simulink model "w3_warplab_buffers"  (Simulink 7.7)
settings: Solver=VariableStepDiscrete  SolverMode=SingleTasking  StartTime=0.0  StopTime=200000  RelTol=1e-3
InitFcn:
  | w3_warplab_buffers_init
StartFcn:
  | w3_warplab_buffers_init
values from neighbouring files (symbols this model uses):
  NumSamps_Rx_IQ = 2^15    (= 32768)    [w3_warplab_buffers_init.m]
  NumSamps_Rx_RSSI = 2^13    (= 8192)    [w3_warplab_buffers_init.m]
  NumSamps_Tx_IQ = 2^15    (= 32768)    [w3_warplab_buffers_init.m]
undefined symbols (not defined in the file or in its folder): gcbh, xlBlockLoadCallback, xlGetNormalizedPeriod
libraries: xbsIndex_r4 x1266, xbsEDKLib_r4 x1
(part 7 of 9)

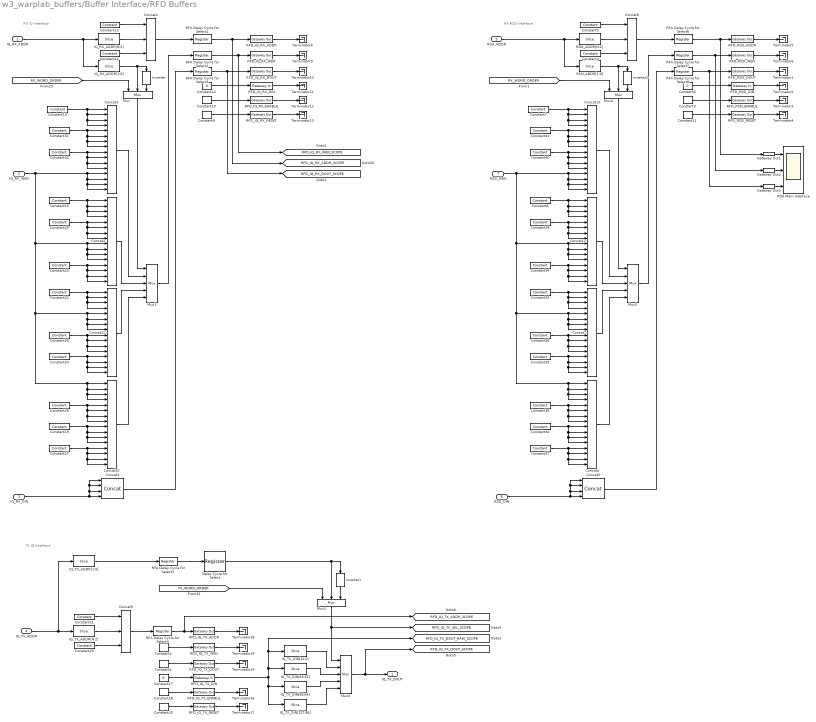
== system w3_warplab_buffers/Buffer Interface/RFD Buffers ==
  note: RX IQ Interface
  note: TX IQ Interface
  note: RX RSSI Interface
  IQ_RX_ADDR : Inport
  IQ_RX_WEN : Inport  Port=2
  IQ_RX_DIN : Inport  Port=3
  IQ_TX_ADDR : Inport  Port=4
  RSSI_ADDR : Inport  Port=5
  RSSI_DIN : Inport  Port=6
  RSSI_WEN : Inport  Port=7
  Concat1 : xbsIndex_r4/Concat  num_inputs=4  dbl_ovrd=off  block_type=concat
  Concat{2..3,6..7,10..13} (8 alike) : xbsIndex_r4/Concat  num_inputs=16  dbl_ovrd=off  block_type=concat
  Concat4 : xbsIndex_r4/Concat  num_inputs=3  dbl_ovrd=off  block_type=concat
  Concat5 : xbsIndex_r4/Concat  num_inputs=4  dbl_ovrd=off  block_type=concat
  Concat8 : xbsIndex_r4/Concat  num_inputs=3  dbl_ovrd=off  block_type=concat
  Concat9 : xbsIndex_r4/Concat  num_inputs=3  dbl_ovrd=off  block_type=concat
  Constant1 : xbsIndex_r4/Constant  const=0  gui_display_data_type=Fixed-point  arith_type=Unsigned  n_bits=128  bin_pt=0  preci_type=Single  exp_width=8  frac_width=24  explicit_period=off  period=1  equ=P=C  opselect=C  inp2=PCIN>>17  opr=+  inp1=P  carry=CIN  dbl_ovrd=off  block_type=constant
      settings: block_version=10.1.2
  Constant10 : xbsIndex_r4/Constant  const=1  gui_display_data_type=Boolean  arith_type=Boolean  n_bits=32  bin_pt=0  preci_type=Single  exp_width=8  frac_width=24  explicit_period=off  period=1  equ=P=C  opselect=C  inp2=PCIN>>17  opr=+  inp1=P  carry=CIN  dbl_ovrd=off  block_type=constant
      settings: block_version=10.1.2
  Constant11 : xbsIndex_r4/Constant  const=0  gui_display_data_type=Boolean  arith_type=Boolean  n_bits=32  bin_pt=0  preci_type=Single  exp_width=8  frac_width=24  explicit_period=off  period=1  equ=P=C  opselect=C  inp2=PCIN>>17  opr=+  inp1=P  carry=CIN  dbl_ovrd=off  block_type=constant
      settings: block_version=10.1.2
  Constant12 : xbsIndex_r4/Constant  const=0  gui_display_data_type=Fixed-point  arith_type=Unsigned  n_bits=4  bin_pt=0  preci_type=Single  exp_width=8  frac_width=24  explicit_period=off  period=1  equ=P=C  opselect=C  inp2=PCIN>>17  opr=+  inp1=P  carry=CIN  dbl_ovrd=off  block_type=constant
  Constant13 : xbsIndex_r4/Constant  const=0  gui_display_data_type=Fixed-point  arith_type=Unsigned  n_bits=30 - ceil(log2(NumSamps_Rx_IQ))  bin_pt=0  preci_type=Single  exp_width=8  frac_width=24  explicit_period=off  period=1  equ=P=C  opselect=C  inp2=PCIN>>17  opr=+  inp1=P  carry=CIN  dbl_ovrd=off  block_type=constant
  Constant14 : Constant  Value=0
  Constant{7..8,15..16,19,22..24,26..41} (24 alike) : xbsIndex_r4/Constant  const=0  gui_display_data_type=Boolean  arith_type=Boolean  n_bits=1  bin_pt=0  preci_type=Single  exp_width=8  frac_width=24  explicit_period=off  period=1  equ=P=C  opselect=C  inp2=PCIN>>17  opr=+  inp1=P  carry=CIN  dbl_ovrd=off  block_type=constant
  Constant17 : Constant  Value=0
  Constant18 : xbsIndex_r4/Constant  const=1  gui_display_data_type=Boolean  arith_type=Boolean  n_bits=32  bin_pt=0  preci_type=Single  exp_width=8  frac_width=24  explicit_period=off  period=1  equ=P=C  opselect=C  inp2=PCIN>>17  opr=+  inp1=P  carry=CIN  dbl_ovrd=off  block_type=constant
      settings: block_version=10.1.2
  Constant2 : xbsIndex_r4/Constant  const=0  gui_display_data_type=Fixed-point  arith_type=Unsigned  n_bits=16  bin_pt=0  preci_type=Single  exp_width=8  frac_width=24  explicit_period=off  period=1  equ=P=C  opselect=C  inp2=PCIN>>17  opr=+  inp1=P  carry=CIN  dbl_ovrd=off  block_type=constant
      settings: block_version=10.1.2
  Constant20 : xbsIndex_r4/Constant  const=0  gui_display_data_type=Fixed-point  arith_type=Unsigned  n_bits=4  bin_pt=0  preci_type=Single  exp_width=8  frac_width=24  explicit_period=off  period=1  equ=P=C  opselect=C  inp2=PCIN>>17  opr=+  inp1=P  carry=CIN  dbl_ovrd=off  block_type=constant
  Constant21 : xbsIndex_r4/Constant  const=0  gui_display_data_type=Fixed-point  arith_type=Unsigned  n_bits=30 - ceil(log2(NumSamps_Tx_IQ))  bin_pt=0  preci_type=Single  exp_width=8  frac_width=24  explicit_period=off  period=1  equ=P=C  opselect=C  inp2=PCIN>>17  opr=+  inp1=P  carry=CIN  dbl_ovrd=off  block_type=constant
  Constant25 : xbsIndex_r4/Constant  const=0  gui_display_data_type=Boolean  arith_type=Boolean  n_bits=32  bin_pt=0  preci_type=Single  exp_width=8  frac_width=24  explicit_period=off  period=1  equ=P=C  opselect=C  inp2=PCIN>>17  opr=+  inp1=P  carry=CIN  dbl_ovrd=off  block_type=constant
      settings: block_version=10.1.2
  Constant3 : xbsIndex_r4/Constant  const=1  gui_display_data_type=Boolean  arith_type=Boolean  n_bits=32  bin_pt=0  preci_type=Single  exp_width=8  frac_width=24  explicit_period=off  period=1  equ=P=C  opselect=C  inp2=PCIN>>17  opr=+  inp1=P  carry=CIN  dbl_ovrd=off  block_type=constant
      settings: block_version=10.1.2
  Constant4 : xbsIndex_r4/Constant  const=0  gui_display_data_type=Fixed-point  arith_type=Unsigned  n_bits=4  bin_pt=0  preci_type=Single  exp_width=8  frac_width=24  explicit_period=off  period=1  equ=P=C  opselect=C  inp2=PCIN>>17  opr=+  inp1=P  carry=CIN  dbl_ovrd=off  block_type=constant
  Constant5 : xbsIndex_r4/Constant  const=0  gui_display_data_type=Fixed-point  arith_type=Unsigned  n_bits=31 - ceil(log2(NumSamps_Rx_RSSI))  bin_pt=0  preci_type=Single  exp_width=8  frac_width=24  explicit_period=off  period=1  equ=P=C  opselect=C  inp2=PCIN>>17  opr=+  inp1=P  carry=CIN  dbl_ovrd=off  block_type=constant
  Constant6 : Constant  Value=0
  Constant9 : xbsIndex_r4/Constant  const=0  gui_display_data_type=Boolean  arith_type=Boolean  n_bits=32  bin_pt=0  preci_type=Single  exp_width=8  frac_width=24  explicit_period=off  period=1  equ=P=C  opselect=C  inp2=PCIN>>17  opr=+  inp1=P  carry=CIN  dbl_ovrd=off  block_type=constant
      settings: block_version=10.1.2
  Delay Cycle for Select : xbsIndex_r4/Register  init=0  rst=off  en=off  dbl_ovrd=off  block_type=register
  Gateway Out1 : xbsIndex_r4/Gateway Out  inherit_from_input=off  hdl_port=off  timing_constraint=None  locs_specified=off  LOCs={}  UseAsDAC=off  DACChannel='1'  block_type=gatewayout
      settings: infoedit="Gateway out block.  Converts Xilinx fixed point inputs into ouputs of type Simulink integer, double, or fixed point.<P><P>Hardware notes:  In hardware these blocks become top level output ports or are discarded, depending on how they are configured."  block_version=10.1.2
  Gateway Out2 : xbsIndex_r4/Gateway Out  inherit_from_input=off  hdl_port=off  timing_constraint=None  locs_specified=off  LOCs={}  UseAsDAC=off  DACChannel='1'  block_type=gatewayout
      settings: infoedit="Gateway out block.  Converts Xilinx fixed point inputs into ouputs of type Simulink integer, double, or fixed point.<P><P>Hardware notes:  In hardware these blocks become top level output ports or are discarded, depending on how they are configured."  block_version=10.1.2
  Gateway Out3 : xbsIndex_r4/Gateway Out  inherit_from_input=off  hdl_port=off  timing_constraint=None  locs_specified=off  LOCs={}  UseAsDAC=off  DACChannel='1'  block_type=gatewayout
      settings: infoedit="Gateway out block.  Converts Xilinx fixed point inputs into ouputs of type Simulink integer, double, or fixed point.<P><P>Hardware notes:  In hardware these blocks become top level output ports or are discarded, depending on how they are configured."  block_version=10.1.2
  IQ_RX_ADDR[1:0] : xbsIndex_r4/Slice  nbits=2  boolean_output=off  mode=Lower Bit Location + Width  bit1=0  base1=MSB of Input  bit0=0  base0=LSB of Input  dbl_ovrd=off  block_type=slice
  IQ_RX_ADDR[N:2] : xbsIndex_r4/Slice  nbits=ceil(log2(NumSamps_Rx_IQ)) - 2  boolean_output=off  mode=Lower Bit Location + Width  bit1=0  base1=MSB of Input  bit0=2  base0=LSB of Input  dbl_ovrd=off  block_type=slice
  IQ_TX_ADDR[1:0] : xbsIndex_r4/Slice  nbits=2  boolean_output=off  mode=Lower Bit Location + Width  bit1=0  base1=MSB of Input  bit0=0  base0=LSB of Input  dbl_ovrd=off  block_type=slice
  IQ_TX_ADDR[N:2] : xbsIndex_r4/Slice  nbits=ceil(log2(NumSamps_Tx_IQ)) - 2  boolean_output=off  mode=Lower Bit Location + Width  bit1=0  base1=MSB of Input  bit0=2  base0=LSB of Input  dbl_ovrd=off  block_type=slice
  IQ_TX_DIN[127:96] : xbsIndex_r4/Slice  nbits=32  boolean_output=off  mode=Lower Bit Location + Width  bit1=0  base1=MSB of Input  bit0=96  base0=LSB of Input  dbl_ovrd=off  block_type=slice
  IQ_TX_DIN[31:0] : xbsIndex_r4/Slice  nbits=32  boolean_output=off  mode=Lower Bit Location + Width  bit1=0  base1=MSB of Input  bit0=0  base0=LSB of Input  dbl_ovrd=off  block_type=slice
  IQ_TX_DIN[63:32] : xbsIndex_r4/Slice  nbits=32  boolean_output=off  mode=Lower Bit Location + Width  bit1=0  base1=MSB of Input  bit0=32  base0=LSB of Input  dbl_ovrd=off  block_type=slice
  IQ_TX_DIN[95:64] : xbsIndex_r4/Slice  nbits=32  boolean_output=off  mode=Lower Bit Location + Width  bit1=0  base1=MSB of Input  bit0=64  base0=LSB of Input  dbl_ovrd=off  block_type=slice
  Inverter : xbsIndex_r4/Inverter  en=off  latency=0  dbl_ovrd=off  block_type=inv
  Inverter1 : xbsIndex_r4/Inverter  en=off  latency=0  dbl_ovrd=off  block_type=inv
  Inverter2 : xbsIndex_r4/Inverter  en=off  latency=0  dbl_ovrd=off  block_type=inv
  Mux : xbsIndex_r4/Mux  inputs=2  en=off  latency=0  precision=Full  arith_type=Unsigned  n_bits=16  bin_pt=14  quantization=Truncate  overflow=Wrap  dbl_ovrd=off  block_type=mux
  Mux1 : xbsIndex_r4/Mux  inputs=4  en=off  latency=0  precision=Full  arith_type=Unsigned  n_bits=16  bin_pt=14  quantization=Truncate  overflow=Wrap  dbl_ovrd=off  block_type=mux
  Mux2 : xbsIndex_r4/Mux  inputs=2  en=off  latency=0  precision=Full  arith_type=Unsigned  n_bits=16  bin_pt=14  quantization=Truncate  overflow=Wrap  dbl_ovrd=off  block_type=mux
  Mux3 : xbsIndex_r4/Mux  inputs=4  en=off  latency=0  precision=Full  arith_type=Unsigned  n_bits=16  bin_pt=14  quantization=Truncate  overflow=Wrap  dbl_ovrd=off  block_type=mux
  Mux4 : xbsIndex_r4/Mux  inputs=2  en=off  latency=0  precision=Full  arith_type=Unsigned  n_bits=16  bin_pt=14  quantization=Truncate  overflow=Wrap  dbl_ovrd=off  block_type=mux
  Mux5 : xbsIndex_r4/Mux  inputs=4  en=off  latency=0  precision=Full  arith_type=Unsigned  n_bits=16  bin_pt=14  quantization=Truncate  overflow=Wrap  dbl_ovrd=off  block_type=mux
  RFA Delay Cycle for Select{1..8} (8 alike) : xbsIndex_r4/Register  init=0  rst=off  en=off  dbl_ovrd=off  block_type=register
  RFD_IQ_RX_ADDR : xbsIndex_r4/Gateway Out  inherit_from_input=off  hdl_port=on  timing_constraint=None  locs_specified=off  LOCs={}  UseAsDAC=off  DACChannel='1'  block_type=gatewayout
  RFD_IQ_RX_DIN : xbsIndex_r4/Gateway In  gui_display_data_type=Fixed-point  arith_type=Unsigned  n_bits=128  bin_pt=0  preci_type=Single  exp_width=8  frac_width=24  quantization="Round  (unbiased: +/- Inf)"  overflow=Saturate  period=1  dbl_ovrd=off  timing_constraint=None  locs_specified=off  LOCs={}  UseAsADC=off  ADCChannel='1'  inherit_from_input=off  hdl_port=on  block_type=gatewayin
  RFD_IQ_RX_DOUT : xbsIndex_r4/Gateway Out  inherit_from_input=off  hdl_port=on  timing_constraint=None  locs_specified=off  LOCs={}  UseAsDAC=off  DACChannel='1'  block_type=gatewayout
  RFD_IQ_RX_ENABLE : xbsIndex_r4/Gateway Out  inherit_from_input=off  hdl_port=on  timing_constraint=None  locs_specified=off  LOCs={}  UseAsDAC=off  DACChannel='1'  block_type=gatewayout
  RFD_IQ_RX_RESET : xbsIndex_r4/Gateway Out  inherit_from_input=off  hdl_port=on  timing_constraint=None  locs_specified=off  LOCs={}  UseAsDAC=off  DACChannel='1'  block_type=gatewayout
  RFD_IQ_RX_WEN : xbsIndex_r4/Gateway Out  inherit_from_input=off  hdl_port=on  timing_constraint=None  locs_specified=off  LOCs={}  UseAsDAC=off  DACChannel='1'  block_type=gatewayout
  RFD_IQ_TX_ADDR : xbsIndex_r4/Gateway Out  inherit_from_input=off  hdl_port=on  timing_constraint=None  locs_specified=off  LOCs={}  UseAsDAC=off  DACChannel='1'  block_type=gatewayout
  RFD_IQ_TX_DIN : xbsIndex_r4/Gateway In  gui_display_data_type=Fixed-point  arith_type=Unsigned  n_bits=128  bin_pt=0  preci_type=Single  exp_width=8  frac_width=24  quantization="Round  (unbiased: +/- Inf)"  overflow=Saturate  period=1  dbl_ovrd=off  timing_constraint=None  locs_specified=off  LOCs={}  UseAsADC=off  ADCChannel='1'  inherit_from_input=off  hdl_port=on  block_type=gatewayin
  RFD_IQ_TX_DOUT : xbsIndex_r4/Gateway Out  inherit_from_input=off  hdl_port=on  timing_constraint=None  locs_specified=off  LOCs={}  UseAsDAC=off  DACChannel='1'  block_type=gatewayout
  RFD_IQ_TX_ENABLE : xbsIndex_r4/Gateway Out  inherit_from_input=off  hdl_port=on  timing_constraint=None  locs_specified=off  LOCs={}  UseAsDAC=off  DACChannel='1'  block_type=gatewayout
  RFD_IQ_TX_RESET : xbsIndex_r4/Gateway Out  inherit_from_input=off  hdl_port=on  timing_constraint=None  locs_specified=off  LOCs={}  UseAsDAC=off  DACChannel='1'  block_type=gatewayout
  RFD_IQ_TX_WEN : xbsIndex_r4/Gateway Out  inherit_from_input=off  hdl_port=on  timing_constraint=None  locs_specified=off  LOCs={}  UseAsDAC=off  DACChannel='1'  block_type=gatewayout
  RFD_RSSI_ADDR : xbsIndex_r4/Gateway Out  inherit_from_input=off  hdl_port=on  timing_constraint=None  locs_specified=off  LOCs={}  UseAsDAC=off  DACChannel='1'  block_type=gatewayout
  RFD_RSSI_DIN : xbsIndex_r4/Gateway In  gui_display_data_type=Fixed-point  arith_type=Unsigned  n_bits=128  bin_pt=0  preci_type=Single  exp_width=8  frac_width=24  quantization="Round  (unbiased: +/- Inf)"  overflow=Saturate  period=1  dbl_ovrd=off  timing_constraint=None  locs_specified=off  LOCs={}  UseAsADC=off  ADCChannel='1'  inherit_from_input=off  hdl_port=on  block_type=gatewayin
  RFD_RSSI_DOUT : xbsIndex_r4/Gateway Out  inherit_from_input=off  hdl_port=on  timing_constraint=None  locs_specified=off  LOCs={}  UseAsDAC=off  DACChannel='1'  block_type=gatewayout
  RFD_RSSI_ENABLE : xbsIndex_r4/Gateway Out  inherit_from_input=off  hdl_port=on  timing_constraint=None  locs_specified=off  LOCs={}  UseAsDAC=off  DACChannel='1'  block_type=gatewayout
  RFD_RSSI_RESET : xbsIndex_r4/Gateway Out  inherit_from_input=off  hdl_port=on  timing_constraint=None  locs_specified=off  LOCs={}  UseAsDAC=off  DACChannel='1'  block_type=gatewayout
  RFD_RSSI_WEN : xbsIndex_r4/Gateway Out  inherit_from_input=off  hdl_port=on  timing_constraint=None  locs_specified=off  LOCs={}  UseAsDAC=off  DACChannel='1'  block_type=gatewayout
  RSSI Mem Interface : Scope  NumInputPorts=3
      settings: TimeRange=70000  YMin=0~0~0  YMax=1~1~1  SaveName=ScopeData6
  RSSI_ADDR[1:0] : xbsIndex_r4/Slice  nbits=2  boolean_output=off  mode=Lower Bit Location + Width  bit1=0  base1=MSB of Input  bit0=0  base0=LSB of Input  dbl_ovrd=off  block_type=slice
  RSSI_ADDR[N:2] : xbsIndex_r4/Slice  nbits=ceil(log2(NumSamps_Rx_RSSI)) - 3  boolean_output=off  mode=Lower Bit Location + Width  bit1=0  base1=MSB of Input  bit0=2  base0=LSB of Input  dbl_ovrd=off  block_type=slice
  Terminator{1..6,8..14,16..19} (17 alike) : Terminator
  IQ_TX_DOUT : Outport
  tag scope: RFD_IQ_RX_ADDR_SCOPE=global, RFD_IQ_RX_DOUT_SCOPE=global, RFD_IQ_RX_WEN_SCOPE=global, RFD_IQ_TX_ADDR_SCOPE=global, RFD_IQ_TX_DOUT_RAW_SCOPE=global, RFD_IQ_TX_DOUT_SCOPE=global, RFD_IQ_TX_SEL_SCOPE=global
  wires:
  IQ_RX_ADDR/1 -> IQ_RX_ADDR[1:0]/1, IQ_RX_ADDR[N:2]/1
  IQ_RX_DIN/1 -> Concat1/4, Concat1/3, Concat1/2, Concat1/1
  RFD_IQ_RX_ADDR/1 -> Terminator8/1
  RFD_IQ_RX_WEN/1 -> Terminator9/1
  RFD_IQ_RX_DOUT/1 -> Terminator10/1
  RFD_IQ_RX_ENABLE/1 -> Terminator12/1
  RFD_IQ_RX_RESET/1 -> Terminator13/1
  RFD_IQ_RX_DIN/1 -> Terminator11/1
  Constant9/1 -> RFD_IQ_RX_RESET/1
  Constant10/1 -> RFD_IQ_RX_ENABLE/1
  Constant14/1 -> RFD_IQ_RX_DIN/1
  Constant13/1 -> Concat4/1
  IQ_RX_ADDR[N:2]/1 -> Concat4/2
  Constant12/1 -> Concat4/3
  Concat4/1 -> RFA Delay Cycle for Select1/1
  Mux1/1 -> RFA Delay Cycle for Select2/1
  IQ_TX_ADDR/1 -> IQ_TX_ADDR[1:0]/1, IQ_TX_ADDR[N:2]/1
  RFD_IQ_TX_ADDR/1 -> Terminator18/1
  RFD_IQ_TX_WEN/1 -> Terminator19/1
  RFD_IQ_TX_DOUT/1 -> Terminator14/1
  RFD_IQ_TX_ENABLE/1 -> Terminator16/1
  RFD_IQ_TX_RESET/1 -> Terminator17/1
  Constant25/1 -> RFD_IQ_TX_RESET/1
  Constant18/1 -> RFD_IQ_TX_ENABLE/1
  Constant21/1 -> Concat9/1
  IQ_TX_ADDR[N:2]/1 -> Concat9/2
  Constant20/1 -> Concat9/3
  Concat9/1 -> RFA Delay Cycle for Select4/1
  Constant2/1 -> RFD_IQ_TX_WEN/1
  Constant1/1 -> RFD_IQ_TX_DOUT/1
  IQ_TX_ADDR[1:0]/1 -> RFA Delay Cycle for Select5/1
  RFD_IQ_TX_DIN/1 -> IQ_TX_DIN[63:32]/1, IQ_TX_DIN[31:0]/1, [RFD_IQ_TX_DOUT_RAW_SCOPE], IQ_TX_DIN[127:96]/1, IQ_TX_DIN[95:64]/1
  IQ_TX_DIN[31:0]/1 -> Mux3/2
  IQ_TX_DIN[63:32]/1 -> Mux3/3
  RFA Delay Cycle for Select1/1 -> RFD_IQ_RX_ADDR/1, [RFD_IQ_RX_ADDR_SCOPE]
  RFA Delay Cycle for Select2/1 -> RFD_IQ_RX_WEN/1, [RFD_IQ_RX_WEN_SCOPE]
  Constant17/1 -> RFD_IQ_TX_DIN/1
  RFA Delay Cycle for Select3/1 -> RFD_IQ_RX_DOUT/1, [RFD_IQ_RX_DOUT_SCOPE]
  Concat1/1 -> RFA Delay Cycle for Select3/1
  RFA Delay Cycle for Select4/1 -> RFD_IQ_TX_ADDR/1, [RFD_IQ_TX_ADDR_SCOPE]
  RFA Delay Cycle for Select5/1 -> Delay Cycle for Select/1
  IQ_RX_ADDR[1:0]/1 -> Inverter/1, Mux/2
  Inverter/1 -> Mux/3
  Mux/1 -> Mux1/1
  Inverter1/1 -> Mux2/3
  Delay Cycle for Select/1 -> Inverter1/1, Mux2/2
  Mux2/1 -> Mux3/1, [RFD_IQ_TX_SEL_SCOPE]
  [RX_WORD_ORDER] -> Mux/1
  Mux3/1 -> IQ_TX_DOUT/1, [RFD_IQ_TX_DOUT_SCOPE]
  RSSI_ADDR/1 -> RSSI_ADDR[1:0]/1, RSSI_ADDR[N:2]/1
  RFD_RSSI_ADDR/1 -> Terminator5/1
  RFD_RSSI_WEN/1 -> Terminator6/1
  RFD_RSSI_DOUT/1 -> Terminator1/1
  RFD_RSSI_ENABLE/1 -> Terminator3/1
  RFD_RSSI_RESET/1 -> Terminator4/1
  RFD_RSSI_DIN/1 -> Terminator2/1
  Constant11/1 -> RFD_RSSI_RESET/1
  Constant3/1 -> RFD_RSSI_ENABLE/1
  Constant6/1 -> RFD_RSSI_DIN/1
  Constant5/1 -> Concat8/1
  RSSI_ADDR[N:2]/1 -> Concat8/2
  Constant4/1 -> Concat8/3
  Concat8/1 -> RFA Delay Cycle for Select6/1
  RFA Delay Cycle for Select6/1 -> RFD_RSSI_ADDR/1, Gateway Out1/1
  RFA Delay Cycle for Select7/1 -> RFD_RSSI_WEN/1, Gateway Out2/1
  RFA Delay Cycle for Select8/1 -> RFD_RSSI_DOUT/1, Gateway Out3/1
  RSSI_ADDR[1:0]/1 -> Inverter2/1, Mux4/2
  Inverter2/1 -> Mux4/3
  Gateway Out1/1 -> RSSI Mem Interface/1
  Gateway Out2/1 -> RSSI Mem Interface/2
  Gateway Out3/1 -> RSSI Mem Interface/3
  Constant15/1 -> Concat3/1, Concat3/2, Concat3/3, Concat3/4
  IQ_RX_WEN/1 -> Concat3/13, Concat3/14, Concat3/15, Concat3/16, Concat2/9, Concat2/10, Concat2/11, Concat2/12, Concat11/5, Concat11/6, Concat11/7, Concat11/8, Concat10/1, Concat10/2, Concat10/3, Concat10/4
  Constant16/1 -> Concat2/1, Concat2/2, Concat2/3, Concat2/4
  Constant23/1 -> Concat2/13, Concat2/14, Concat2/15, Concat2/16
  Constant22/1 -> Concat11/3, Concat11/4, Concat11/2, Concat11/1
  Constant24/1 -> Concat11/15, Concat11/16, Concat11/14, Concat11/13
  Constant26/1 -> Concat11/11, Concat11/12, Concat11/10, Concat11/9
  Constant27/1 -> Concat10/15, Concat10/16, Concat10/14, Concat10/13
  Constant19/1 -> Concat10/11, Concat10/12, Concat10/10, Concat10/9
  Constant28/1 -> Concat10/7, Concat10/8, Concat10/6, Concat10/5
  Constant29/1 -> Concat2/7, Concat2/8, Concat2/6, Concat2/5
  Constant30/1 -> Concat3/11, Concat3/12, Concat3/10, Concat3/9
  Constant31/1 -> Concat3/7, Concat3/8, Concat3/6, Concat3/5
  Concat3/1 -> Mux1/2
  Concat2/1 -> Mux1/3
  Concat11/1 -> Mux1/4
  Concat10/1 -> Mux1/5
  [RX_WORD_ORDER] -> Mux4/1
  [TX_WORD_ORDER] -> Mux2/1
  RSSI_DIN/1 -> Concat5/4, Concat5/3, Concat5/2, Concat5/1
  Mux5/1 -> RFA Delay Cycle for Select7/1
  Concat5/1 -> RFA Delay Cycle for Select8/1
  Mux4/1 -> Mux5/1
  Constant7/1 -> Concat13/1, Concat13/2, Concat13/3, Concat13/4
  RSSI_WEN/1 -> Concat13/13, Concat13/14, Concat13/15, Concat13/16, Concat12/9, Concat12/10, Concat12/11, Concat12/12, Concat7/5, Concat7/6, Concat7/7, Concat7/8, Concat6/1, Concat6/2, Concat6/3, Concat6/4
  Constant8/1 -> Concat12/1, Concat12/2, Concat12/3, Concat12/4
  Constant34/1 -> Concat12/13, Concat12/14, Concat12/15, Concat12/16
  Constant33/1 -> Concat7/3, Concat7/4, Concat7/2, Concat7/1
  Constant35/1 -> Concat7/15, Concat7/16, Concat7/14, Concat7/13
  Constant36/1 -> Concat7/11, Concat7/12, Concat7/10, Concat7/9
  Constant37/1 -> Concat6/15, Concat6/16, Concat6/14, Concat6/13
  Constant32/1 -> Concat6/11, Concat6/12, Concat6/10, Concat6/9
  Constant38/1 -> Concat6/7, Concat6/8, Concat6/6, Concat6/5
  Constant39/1 -> Concat12/7, Concat12/8, Concat12/6, Concat12/5
  Constant40/1 -> Concat13/11, Concat13/12, Concat13/10, Concat13/9
  Constant41/1 -> Concat13/7, Concat13/8, Concat13/6, Concat13/5
  Concat13/1 -> Mux5/2
  Concat12/1 -> Mux5/3
  Concat7/1 -> Mux5/4
  Concat6/1 -> Mux5/5
  IQ_TX_DIN[95:64]/1 -> Mux3/4
  IQ_TX_DIN[127:96]/1 -> Mux3/5

== system w3_warplab_buffers/Memory-mapped Registers/COUNTER_RESET ==
  32b : Inport
  Convert{1..8} (8 alike) : xbsIndex_r4/Convert  gui_display_data_type=Boolean  arith_type=Boolean  n_bits=32  bin_pt=0  float_type=Single  exp_bits=8  fraction_bits=24  quantization=Truncate  overflow=Wrap  en=off  latency=0  dbl_ovrd=off  pipeline=off  block_type=convert
      settings: block_version=8.2
  Posedge : Subsystem
  Posedge1 : Subsystem
  Posedge2 : Subsystem
  Posedge3 : Subsystem
  Posedge4 : Subsystem
  Posedge5 : Subsystem
  Posedge6 : Subsystem
  Posedge7 : Subsystem
  b[0] : xbsIndex_r4/Slice  nbits=1  boolean_output=off  mode=Lower Bit Location + Width  bit1=0  base1=MSB of Input  bit0=0  base0=LSB of Input  dbl_ovrd=off  block_type=slice
  b[10] : xbsIndex_r4/Slice  nbits=1  boolean_output=off  mode=Lower Bit Location + Width  bit1=0  base1=MSB of Input  bit0=2  base0=LSB of Input  dbl_ovrd=off  block_type=slice
  b[11] : xbsIndex_r4/Slice  nbits=1  boolean_output=off  mode=Lower Bit Location + Width  bit1=0  base1=MSB of Input  bit0=3  base0=LSB of Input  dbl_ovrd=off  block_type=slice
  b[1] : xbsIndex_r4/Slice  nbits=1  boolean_output=off  mode=Lower Bit Location + Width  bit1=0  base1=MSB of Input  bit0=1  base0=LSB of Input  dbl_ovrd=off  block_type=slice
  b[2] : xbsIndex_r4/Slice  nbits=1  boolean_output=off  mode=Lower Bit Location + Width  bit1=0  base1=MSB of Input  bit0=2  base0=LSB of Input  dbl_ovrd=off  block_type=slice
  b[3] : xbsIndex_r4/Slice  nbits=1  boolean_output=off  mode=Lower Bit Location + Width  bit1=0  base1=MSB of Input  bit0=3  base0=LSB of Input  dbl_ovrd=off  block_type=slice
  b[8] : xbsIndex_r4/Slice  nbits=1  boolean_output=off  mode=Lower Bit Location + Width  bit1=0  base1=MSB of Input  bit0=0  base0=LSB of Input  dbl_ovrd=off  block_type=slice
  b[9] : xbsIndex_r4/Slice  nbits=1  boolean_output=off  mode=Lower Bit Location + Width  bit1=0  base1=MSB of Input  bit0=1  base0=LSB of Input  dbl_ovrd=off  block_type=slice
  RFA_TX : Outport
  RFB_TX : Outport  Port=2
  RFC_TX : Outport  Port=3
  RFD_TX : Outport  Port=4
  RFA_RX : Outport  Port=5
  RFB_RX : Outport  Port=6
  RFC_RX : Outport  Port=7
  RFD_RX : Outport  Port=8
  wires:
  b[0]/1 -> Posedge/1(D)
  b[1]/1 -> Posedge1/1(D)
  b[2]/1 -> Posedge2/1(D)
  b[3]/1 -> Posedge3/1(D)
  32b/1 -> b[0]/1, b[1]/1, b[2]/1, b[3]/1, b[8]/1, b[9]/1, b[10]/1, b[11]/1
  b[8]/1 -> Posedge4/1(D)
  b[9]/1 -> Posedge5/1(D)
  b[10]/1 -> Posedge6/1(D)
  b[11]/1 -> Posedge7/1(D)
  Posedge/1(Q) -> Convert4/1
  Posedge1/1(Q) -> Convert1/1
  Posedge2/1(Q) -> Convert2/1
  Posedge3/1(Q) -> Convert3/1
  Posedge4/1(Q) -> Convert5/1
  Posedge5/1(Q) -> Convert6/1
  Posedge6/1(Q) -> Convert7/1
  Posedge7/1(Q) -> Convert8/1
  Convert4/1 -> RFA_TX/1
  Convert1/1 -> RFB_TX/1
  Convert2/1 -> RFC_TX/1
  Convert3/1 -> RFD_TX/1
  Convert5/1 -> RFA_RX/1
  Convert6/1 -> RFB_RX/1
  Convert7/1 -> RFC_RX/1
  Convert8/1 -> RFD_RX/1

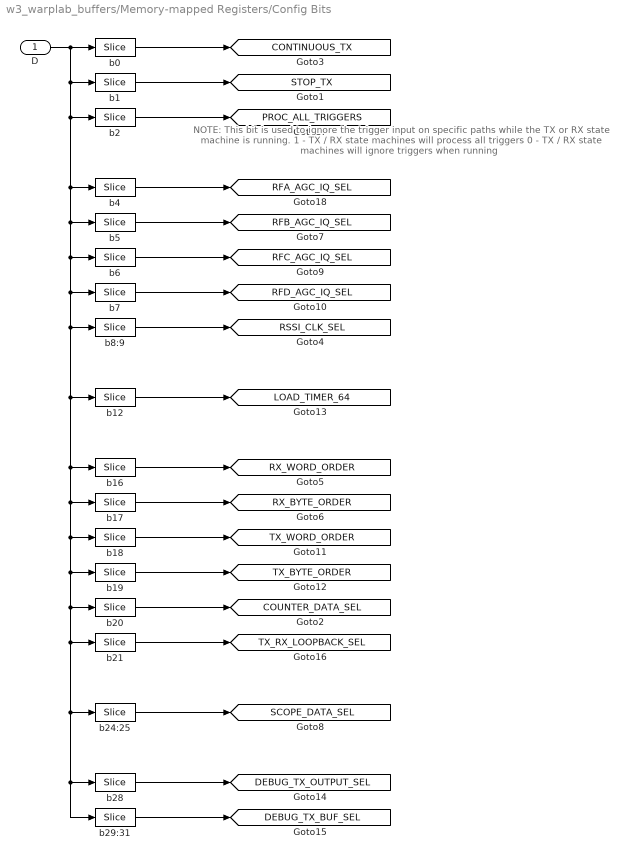
== system w3_warplab_buffers/Memory-mapped Registers/Config Bits ==
  note: NOTE:  This bit is used to ignore the trigger input on specific paths while the TX or RX state machine is running.
      |       1  -   TX / RX state machines will process all triggers
      |       0  -   TX / RX state machines will ignore triggers when running
  D : Inport
  b0 : xbsIndex_r4/Slice  nbits=1  boolean_output=off  mode=Lower Bit Location + Width  bit1=0  base1=MSB of Input  bit0=0  base0=LSB of Input  dbl_ovrd=off  block_type=slice
  b1 : xbsIndex_r4/Slice  nbits=1  boolean_output=off  mode=Lower Bit Location + Width  bit1=0  base1=MSB of Input  bit0=1  base0=LSB of Input  dbl_ovrd=off  block_type=slice
  b12 : xbsIndex_r4/Slice  nbits=1  boolean_output=off  mode=Lower Bit Location + Width  bit1=0  base1=MSB of Input  bit0=12  base0=LSB of Input  dbl_ovrd=off  block_type=slice
  b16 : xbsIndex_r4/Slice  nbits=1  boolean_output=off  mode=Lower Bit Location + Width  bit1=0  base1=MSB of Input  bit0=16  base0=LSB of Input  dbl_ovrd=off  block_type=slice
  b17 : xbsIndex_r4/Slice  nbits=1  boolean_output=off  mode=Lower Bit Location + Width  bit1=0  base1=MSB of Input  bit0=17  base0=LSB of Input  dbl_ovrd=off  block_type=slice
  b18 : xbsIndex_r4/Slice  nbits=1  boolean_output=off  mode=Lower Bit Location + Width  bit1=0  base1=MSB of Input  bit0=18  base0=LSB of Input  dbl_ovrd=off  block_type=slice
  b19 : xbsIndex_r4/Slice  nbits=1  boolean_output=off  mode=Lower Bit Location + Width  bit1=0  base1=MSB of Input  bit0=19  base0=LSB of Input  dbl_ovrd=off  block_type=slice
  b2 : xbsIndex_r4/Slice  nbits=1  boolean_output=off  mode=Lower Bit Location + Width  bit1=0  base1=MSB of Input  bit0=2  base0=LSB of Input  dbl_ovrd=off  block_type=slice
  b20 : xbsIndex_r4/Slice  nbits=1  boolean_output=off  mode=Lower Bit Location + Width  bit1=0  base1=MSB of Input  bit0=20  base0=LSB of Input  dbl_ovrd=off  block_type=slice
  b21 : xbsIndex_r4/Slice  nbits=1  boolean_output=off  mode=Lower Bit Location + Width  bit1=0  base1=MSB of Input  bit0=21  base0=LSB of Input  dbl_ovrd=off  block_type=slice
  b24:25 : xbsIndex_r4/Slice  nbits=2  boolean_output=off  mode=Lower Bit Location + Width  bit1=0  base1=MSB of Input  bit0=24  base0=LSB of Input  dbl_ovrd=off  block_type=slice
  b28 : xbsIndex_r4/Slice  nbits=1  boolean_output=off  mode=Lower Bit Location + Width  bit1=0  base1=MSB of Input  bit0=28  base0=LSB of Input  dbl_ovrd=off  block_type=slice
  b29:31 : xbsIndex_r4/Slice  nbits=3  boolean_output=off  mode=Lower Bit Location + Width  bit1=0  base1=MSB of Input  bit0=29  base0=LSB of Input  dbl_ovrd=off  block_type=slice
  b4 : xbsIndex_r4/Slice  nbits=1  boolean_output=off  mode=Lower Bit Location + Width  bit1=0  base1=MSB of Input  bit0=4  base0=LSB of Input  dbl_ovrd=off  block_type=slice
  b5 : xbsIndex_r4/Slice  nbits=1  boolean_output=off  mode=Lower Bit Location + Width  bit1=0  base1=MSB of Input  bit0=5  base0=LSB of Input  dbl_ovrd=off  block_type=slice
  b6 : xbsIndex_r4/Slice  nbits=1  boolean_output=off  mode=Lower Bit Location + Width  bit1=0  base1=MSB of Input  bit0=6  base0=LSB of Input  dbl_ovrd=off  block_type=slice
  b7 : xbsIndex_r4/Slice  nbits=1  boolean_output=off  mode=Lower Bit Location + Width  bit1=0  base1=MSB of Input  bit0=7  base0=LSB of Input  dbl_ovrd=off  block_type=slice
  b8:9 : xbsIndex_r4/Slice  nbits=2  boolean_output=off  mode=Lower Bit Location + Width  bit1=0  base1=MSB of Input  bit0=8  base0=LSB of Input  dbl_ovrd=off  block_type=slice
  tag scope: CONTINUOUS_TX=global, COUNTER_DATA_SEL=global, DEBUG_TX_BUF_SEL=global, DEBUG_TX_OUTPUT_SEL=global, LOAD_TIMER_64=global, PROC_ALL_TRIGGERS=global, RFA_AGC_IQ_SEL=global, RFB_AGC_IQ_SEL=global, RFC_AGC_IQ_SEL=global, RFD_AGC_IQ_SEL=global, RSSI_CLK_SEL=global, RX_BYTE_ORDER=global, RX_WORD_ORDER=global, SCOPE_DATA_SEL=global, STOP_TX=global, TX_BYTE_ORDER=global, TX_RX_LOOPBACK_SEL=global, TX_WORD_ORDER=global
  wires:
  D/1 -> b1/1, b4/1, b5/1, b6/1, b17/1, b8:9/1, b18/1, b20/1, b24:25/1, b28/1, b29:31/1, b21/1, b19/1, b12/1, b16/1, b7/1, b2/1, b0/1
  b0/1 -> [CONTINUOUS_TX]
  b1/1 -> [STOP_TX]
  b4/1 -> [RFA_AGC_IQ_SEL]
  b17/1 -> [RX_BYTE_ORDER]
  b8:9/1 -> [RSSI_CLK_SEL]
  b16/1 -> [RX_WORD_ORDER]
  b20/1 -> [COUNTER_DATA_SEL]
  b24:25/1 -> [SCOPE_DATA_SEL]
  b5/1 -> [RFB_AGC_IQ_SEL]
  b6/1 -> [RFC_AGC_IQ_SEL]
  b7/1 -> [RFD_AGC_IQ_SEL]
  b19/1 -> [TX_BYTE_ORDER]
  b18/1 -> [TX_WORD_ORDER]
  b12/1 -> [LOAD_TIMER_64]
  b28/1 -> [DEBUG_TX_OUTPUT_SEL]
  b29:31/1 -> [DEBUG_TX_BUF_SEL]
  b21/1 -> [TX_RX_LOOPBACK_SEL]
  b2/1 -> [PROC_ALL_TRIGGERS]

== system w3_warplab_buffers/Memory-mapped Registers/Posedge ==
  D : Inport
  Delay : xbsIndex_r4/Delay  rst=off  infoeditControl=Selection of Reset will increase slice count due to use of real FFs and instead of SRLs  en=off  latency=1  dbl_ovrd=off  reg_retiming=off  block_type=delay
      settings: infoedit=Hardware notes: A delay line is a chain, each link of which is an SRL16 followed by a flip-flop. If register retiming is enabled, the delay line is a chain of flip-flops.  block_version=8.2
  Inverter : xbsIndex_r4/Inverter  en=off  latency=0  dbl_ovrd=off  block_type=inv
      settings: block_version=8.2
  Logical : xbsIndex_r4/Logical  logical_function=AND  inputs=2  en=off  latency=0  precision=Full  arith_type=Unsigned  n_bits=16  bin_pt=0  align_bp=on  dbl_ovrd=off  block_type=logical
      settings: block_version=8.2
  Q : Outport
  wires:
  D/1 -> Inverter/1, Logical/1
  Inverter/1 -> Delay/1
  Delay/1 -> Logical/2
  Logical/1 -> Q/1

== system w3_warplab_buffers/Memory-mapped Registers/Posedge1 ==
  D : Inport
  Delay : xbsIndex_r4/Delay  rst=off  infoeditControl=Selection of Reset will increase slice count due to use of real FFs and instead of SRLs  en=off  latency=1  dbl_ovrd=off  reg_retiming=off  block_type=delay
      settings: infoedit=Hardware notes: A delay line is a chain, each link of which is an SRL16 followed by a flip-flop. If register retiming is enabled, the delay line is a chain of flip-flops.  block_version=8.2
  Inverter : xbsIndex_r4/Inverter  en=off  latency=0  dbl_ovrd=off  block_type=inv
      settings: block_version=8.2
  Logical : xbsIndex_r4/Logical  logical_function=AND  inputs=2  en=off  latency=0  precision=Full  arith_type=Unsigned  n_bits=16  bin_pt=0  align_bp=on  dbl_ovrd=off  block_type=logical
      settings: block_version=8.2
  Q : Outport
  wires:
  D/1 -> Inverter/1, Logical/1
  Inverter/1 -> Delay/1
  Delay/1 -> Logical/2
  Logical/1 -> Q/1

== system w3_warplab_buffers/Memory-mapped Registers/Posedge2 ==
  D : Inport
  Delay : xbsIndex_r4/Delay  rst=off  infoeditControl=Selection of Reset will increase slice count due to use of real FFs and instead of SRLs  en=off  latency=1  dbl_ovrd=off  reg_retiming=off  block_type=delay
      settings: infoedit=Hardware notes: A delay line is a chain, each link of which is an SRL16 followed by a flip-flop. If register retiming is enabled, the delay line is a chain of flip-flops.  block_version=8.2
  Inverter : xbsIndex_r4/Inverter  en=off  latency=0  dbl_ovrd=off  block_type=inv
      settings: block_version=8.2
  Logical : xbsIndex_r4/Logical  logical_function=AND  inputs=2  en=off  latency=0  precision=Full  arith_type=Unsigned  n_bits=16  bin_pt=0  align_bp=on  dbl_ovrd=off  block_type=logical
      settings: block_version=8.2
  Q : Outport
  wires:
  D/1 -> Inverter/1, Logical/1
  Inverter/1 -> Delay/1
  Delay/1 -> Logical/2
  Logical/1 -> Q/1

== system w3_warplab_buffers/Memory-mapped Registers/Posedge3 ==
  D : Inport
  Delay : xbsIndex_r4/Delay  rst=off  infoeditControl=Selection of Reset will increase slice count due to use of real FFs and instead of SRLs  en=off  latency=1  dbl_ovrd=off  reg_retiming=off  block_type=delay
      settings: infoedit=Hardware notes: A delay line is a chain, each link of which is an SRL16 followed by a flip-flop. If register retiming is enabled, the delay line is a chain of flip-flops.  block_version=8.2
  Inverter : xbsIndex_r4/Inverter  en=off  latency=0  dbl_ovrd=off  block_type=inv
      settings: block_version=8.2
  Logical : xbsIndex_r4/Logical  logical_function=AND  inputs=2  en=off  latency=0  precision=Full  arith_type=Unsigned  n_bits=16  bin_pt=0  align_bp=on  dbl_ovrd=off  block_type=logical
      settings: block_version=8.2
  Q : Outport
  wires:
  D/1 -> Inverter/1, Logical/1
  Inverter/1 -> Delay/1
  Delay/1 -> Logical/2
  Logical/1 -> Q/1

== system w3_warplab_buffers/Memory-mapped Registers/Posedge4 ==
  D : Inport
  Delay : xbsIndex_r4/Delay  rst=off  infoeditControl=Selection of Reset will increase slice count due to use of real FFs and instead of SRLs  en=off  latency=1  dbl_ovrd=off  reg_retiming=off  block_type=delay
      settings: infoedit=Hardware notes: A delay line is a chain, each link of which is an SRL16 followed by a flip-flop. If register retiming is enabled, the delay line is a chain of flip-flops.  block_version=8.2
  Inverter : xbsIndex_r4/Inverter  en=off  latency=0  dbl_ovrd=off  block_type=inv
      settings: block_version=8.2
  Logical : xbsIndex_r4/Logical  logical_function=AND  inputs=2  en=off  latency=0  precision=Full  arith_type=Unsigned  n_bits=16  bin_pt=0  align_bp=on  dbl_ovrd=off  block_type=logical
      settings: block_version=8.2
  Q : Outport
  wires:
  D/1 -> Inverter/1, Logical/1
  Inverter/1 -> Delay/1
  Delay/1 -> Logical/2
  Logical/1 -> Q/1

== system w3_warplab_buffers/Memory-mapped Registers/Posedge5 ==
  D : Inport
  Delay : xbsIndex_r4/Delay  rst=off  infoeditControl=Selection of Reset will increase slice count due to use of real FFs and instead of SRLs  en=off  latency=1  dbl_ovrd=off  reg_retiming=off  block_type=delay
      settings: infoedit=Hardware notes: A delay line is a chain, each link of which is an SRL16 followed by a flip-flop. If register retiming is enabled, the delay line is a chain of flip-flops.  block_version=8.2
  Inverter : xbsIndex_r4/Inverter  en=off  latency=0  dbl_ovrd=off  block_type=inv
      settings: block_version=8.2
  Logical : xbsIndex_r4/Logical  logical_function=AND  inputs=2  en=off  latency=0  precision=Full  arith_type=Unsigned  n_bits=16  bin_pt=0  align_bp=on  dbl_ovrd=off  block_type=logical
      settings: block_version=8.2
  Q : Outport
  wires:
  D/1 -> Inverter/1, Logical/1
  Inverter/1 -> Delay/1
  Delay/1 -> Logical/2
  Logical/1 -> Q/1

== system w3_warplab_buffers/Memory-mapped Registers/Posedge6 ==
  D : Inport
  Delay : xbsIndex_r4/Delay  rst=off  infoeditControl=Selection of Reset will increase slice count due to use of real FFs and instead of SRLs  en=off  latency=1  dbl_ovrd=off  reg_retiming=off  block_type=delay
      settings: infoedit=Hardware notes: A delay line is a chain, each link of which is an SRL16 followed by a flip-flop. If register retiming is enabled, the delay line is a chain of flip-flops.  block_version=8.2
  Inverter : xbsIndex_r4/Inverter  en=off  latency=0  dbl_ovrd=off  block_type=inv
      settings: block_version=8.2
  Logical : xbsIndex_r4/Logical  logical_function=AND  inputs=2  en=off  latency=0  precision=Full  arith_type=Unsigned  n_bits=16  bin_pt=0  align_bp=on  dbl_ovrd=off  block_type=logical
      settings: block_version=8.2
  Q : Outport
  wires:
  D/1 -> Inverter/1, Logical/1
  Inverter/1 -> Delay/1
  Delay/1 -> Logical/2
  Logical/1 -> Q/1

== system w3_warplab_buffers/Memory-mapped Registers/Posedge7 ==
  D : Inport
  Delay : xbsIndex_r4/Delay  rst=off  infoeditControl=Selection of Reset will increase slice count due to use of real FFs and instead of SRLs  en=off  latency=1  dbl_ovrd=off  reg_retiming=off  block_type=delay
      settings: infoedit=Hardware notes: A delay line is a chain, each link of which is an SRL16 followed by a flip-flop. If register retiming is enabled, the delay line is a chain of flip-flops.  block_version=8.2
  Inverter : xbsIndex_r4/Inverter  en=off  latency=0  dbl_ovrd=off  block_type=inv
      settings: block_version=8.2
  Logical : xbsIndex_r4/Logical  logical_function=AND  inputs=2  en=off  latency=0  precision=Full  arith_type=Unsigned  n_bits=16  bin_pt=0  align_bp=on  dbl_ovrd=off  block_type=logical
      settings: block_version=8.2
  Q : Outport
  wires:
  D/1 -> Inverter/1, Logical/1
  Inverter/1 -> Delay/1
  Delay/1 -> Logical/2
  Logical/1 -> Q/1

== system w3_warplab_buffers/Memory-mapped Registers/RF RUNNING ==
   {1..8} (8 alike) : xbsIndex_r4/Logical  logical_function=AND  inputs=2  en=off  latency=0  precision=Full  arith_type=Unsigned  n_bits=16  bin_pt=0  align_bp=on  dbl_ovrd=off  block_type=logical
      settings: block_version=9.1.01
  Convert{2..3,5..10} (8 alike) : xbsIndex_r4/Convert  gui_display_data_type=Boolean  arith_type=Boolean  n_bits=32  bin_pt=0  float_type=Single  exp_bits=8  fraction_bits=24  quantization=Truncate  overflow=Wrap  en=off  latency=0  dbl_ovrd=off  pipeline=off  block_type=convert
      settings: block_version=8.2
  RFA_TX : Outport
  RFB_TX : Outport  Port=2
  RFC_TX : Outport  Port=3
  RFD_TX : Outport  Port=4
  RFA_RX : Outport  Port=5
  RFB_RX : Outport  Port=6
  RFC_RX : Outport  Port=7
  RFD_RX : Outport  Port=8
  wires:
  " 2"/1 -> RFD_TX/1
  " 3"/1 -> RFB_TX/1
  " 4"/1 -> RFA_TX/1
  " 1"/1 -> RFC_TX/1
  " 6"/1 -> RFD_RX/1
  " 5"/1 -> RFC_RX/1
  " 7"/1 -> RFB_RX/1
  " 8"/1 -> RFA_RX/1
  [TX_RUNNING] -> " 4"/2, " 3"/2, " 1"/2, " 2"/2
  [RX_RUNNING] -> " 7"/2, " 5"/2, " 6"/2, " 8"/2
  Convert2/1 -> " 6"/1
  Convert3/1 -> " 5"/1
  Convert5/1 -> " 7"/1
  Convert6/1 -> " 8"/1
  Convert7/1 -> " 2"/1
  Convert8/1 -> " 1"/1
  Convert9/1 -> " 3"/1
  Convert10/1 -> " 4"/1
  [RFA_TX_BUF_EN] -> Convert10/1
  [RFB_TX_BUF_EN] -> Convert9/1
  [RFC_TX_BUF_EN] -> Convert8/1
  [RFD_TX_BUF_EN] -> Convert7/1
  [RFA_RX_BUF_EN] -> Convert6/1
  [RFB_RX_BUF_EN] -> Convert5/1
  [RFC_RX_BUF_EN] -> Convert3/1
  [RFD_RX_BUF_EN] -> Convert2/1

== system w3_warplab_buffers/Memory-mapped Registers/RFx Sel ==
  32b : Inport
  b0 : xbsIndex_r4/Slice  nbits=1  boolean_output=off  mode=Lower Bit Location + Width  bit1=0  base1=MSB of Input  bit0=0  base0=LSB of Input  dbl_ovrd=off  block_type=slice
  b1 : xbsIndex_r4/Slice  nbits=1  boolean_output=off  mode=Lower Bit Location + Width  bit1=0  base1=MSB of Input  bit0=1  base0=LSB of Input  dbl_ovrd=off  block_type=slice
  b2 : xbsIndex_r4/Slice  nbits=1  boolean_output=off  mode=Lower Bit Location + Width  bit1=1  base1=MSB of Input  bit0=2  base0=LSB of Input  dbl_ovrd=off  block_type=slice
  b3 : xbsIndex_r4/Slice  nbits=1  boolean_output=off  mode=Lower Bit Location + Width  bit1=1  base1=MSB of Input  bit0=3  base0=LSB of Input  dbl_ovrd=off  block_type=slice
  A : Outport
  B : Outport  Port=2
  C : Outport  Port=3
  D : Outport  Port=4
  wires:
  32b/1 -> b0/1, b1/1, b2/1, b3/1
  b3/1 -> D/1
  b2/1 -> C/1
  b1/1 -> B/1
  b0/1 -> A/1

== system w3_warplab_buffers/Memory-mapped Registers/RFx Sel2 ==
  32b : Inport
  b0 : xbsIndex_r4/Slice  nbits=1  boolean_output=off  mode=Lower Bit Location + Width  bit1=0  base1=MSB of Input  bit0=0  base0=LSB of Input  dbl_ovrd=off  block_type=slice
  b1 : xbsIndex_r4/Slice  nbits=1  boolean_output=off  mode=Lower Bit Location + Width  bit1=0  base1=MSB of Input  bit0=1  base0=LSB of Input  dbl_ovrd=off  block_type=slice
  b2 : xbsIndex_r4/Slice  nbits=1  boolean_output=off  mode=Lower Bit Location + Width  bit1=1  base1=MSB of Input  bit0=2  base0=LSB of Input  dbl_ovrd=off  block_type=slice
  b3 : xbsIndex_r4/Slice  nbits=1  boolean_output=off  mode=Lower Bit Location + Width  bit1=1  base1=MSB of Input  bit0=3  base0=LSB of Input  dbl_ovrd=off  block_type=slice
  A : Outport
  B : Outport  Port=2
  C : Outport  Port=3
  D : Outport  Port=4
  wires:
  32b/1 -> b0/1, b1/1, b2/1, b3/1
  b3/1 -> D/1
  b2/1 -> C/1
  b1/1 -> B/1
  b0/1 -> A/1

== system w3_warplab_buffers/Memory-mapped Registers/Timer64 ==
  note: NOTE: Counter is set to use 40 MHz clock input. If that changes, please modify the "usec Pulse" block.
  Load : Inport
  Load MSB : Inport  Port=2
  Load LSB : Inport  Port=3
  32LSB : xbsIndex_r4/Slice  nbits=32  boolean_output=off  mode=Lower Bit Location + Width  bit1=0  base1=MSB of Input  bit0=0  base0=LSB of Input  dbl_ovrd=off  block_type=slice
      settings: block_version=VER_STRING_GOES_HERE
  32MSB : xbsIndex_r4/Slice  nbits=32  boolean_output=off  mode=Upper Bit Location + Width  bit1=0  base1=MSB of Input  bit0=0  base0=LSB of Input  dbl_ovrd=off  block_type=slice
      settings: block_version=VER_STRING_GOES_HERE
  Concat : xbsIndex_r4/Concat  num_inputs=2  dbl_ovrd=off  block_type=concat
  Convert4 : xbsIndex_r4/Convert  gui_display_data_type=Boolean  arith_type=Boolean  n_bits=32  bin_pt=0  float_type=Single  exp_bits=8  fraction_bits=24  quantization=Truncate  overflow=Wrap  en=off  latency=0  dbl_ovrd=off  pipeline=off  block_type=convert
      settings: block_version=8.2
  Counter : Scope  NumInputPorts=7
      settings: TimeRange=70000  YMin=0~0~0~0~0~-5~-5  YMax=1~1~1~100~20000~5~5  SaveName=ScopeData7
  Gateway Out{1..7} (7 alike) : xbsIndex_r4/Gateway Out  inherit_from_input=off  hdl_port=off  timing_constraint=None  locs_specified=off  LOCs={}  UseAsDAC=off  DACChannel='1'  block_type=gatewayout
      settings: infoedit="Gateway out block.  Converts Xilinx fixed point inputs into ouputs of type Simulink integer, double, or fixed point.<P><P>Hardware notes:  In hardware these blocks become top level output ports or are discarded, depending on how they are configured."  block_version=10.1.2
  Logical : xbsIndex_r4/Logical  logical_function=OR  inputs=2  en=off  latency=0  precision=Full  arith_type=Unsigned  n_bits=16  bin_pt=0  align_bp=on  dbl_ovrd=off  block_type=logical
  Microsecond Counter : xbsIndex_r4/Counter  cnt_type=Free Running  cnt_to=Inf  operation=Up  start_count=0  cnt_by_val=1  arith_type=Unsigned  n_bits=64  bin_pt=0  load_pin=on  rst=off  en=on  explicit_period=off  period=1  dbl_ovrd=off  use_behavioral_HDL=off  implementation=Fabric  block_type=counter
  Posedge2 : Subsystem
  Register{,1..3} (4 alike) : xbsIndex_r4/Register  init=0  rst=off  en=off  dbl_ovrd=off  block_type=register
  usec Pulse : Subsystem
  CNT_MSB : Outport
  CNT_LSB : Outport  Port=2
  wires:
  Microsecond Counter/1 -> 32LSB/1, 32MSB/1, Gateway Out5/1
  32LSB/1 -> Register2/1
  32MSB/1 -> Register1/1
  Register/1 -> CNT_MSB/1, Gateway Out6/1
  Register1/1 -> Register/1
  Register2/1 -> Register3/1
  Register3/1 -> CNT_LSB/1, Gateway Out7/1
  Logical/1 -> Microsecond Counter/3
  usec Pulse/1(uSec) -> Logical/2, Gateway Out4/1
  Load LSB/1 -> Concat/2, Gateway Out3/1
  Load MSB/1 -> Concat/1, Gateway Out2/1
  Concat/1 -> Microsecond Counter/2
  Load/1 -> Posedge2/1(D), Gateway Out1/1
  Posedge2/1(Q) -> Convert4/1
  Convert4/1 -> Microsecond Counter/1, Logical/1, usec Pulse/1(Rst)
  Gateway Out5/1 -> Counter/5
  Gateway Out4/1 -> Counter/4
  Gateway Out3/1 -> Counter/3
  Gateway Out2/1 -> Counter/2
  Gateway Out1/1 -> Counter/1
  Gateway Out7/1 -> Counter/7
  Gateway Out6/1 -> Counter/6

== system w3_warplab_buffers/RFA Rx Buffers/I/Q Buffer ==
  Addr : Inport
  I/Q_32b : Inport  Port=2
  WE : Inport  Port=3
  8LSB+0 : xbsIndex_r4/Slice  nbits=8  boolean_output=off  mode=Lower Bit Location + Width  bit1=0  base1=MSB of Input  bit0=0  base0=LSB of Input  dbl_ovrd=off  block_type=slice
  8LSB+16 : xbsIndex_r4/Slice  nbits=8  boolean_output=off  mode=Lower Bit Location + Width  bit1=0  base1=MSB of Input  bit0=16  base0=LSB of Input  dbl_ovrd=off  block_type=slice
  8LSB+24 : xbsIndex_r4/Slice  nbits=8  boolean_output=off  mode=Lower Bit Location + Width  bit1=0  base1=MSB of Input  bit0=24  base0=LSB of Input  dbl_ovrd=off  block_type=slice
  8LSB+8 : xbsIndex_r4/Slice  nbits=8  boolean_output=off  mode=Lower Bit Location + Width  bit1=0  base1=MSB of Input  bit0=8  base0=LSB of Input  dbl_ovrd=off  block_type=slice
  Concat : xbsIndex_r4/Concat  num_inputs=4  dbl_ovrd=off  block_type=concat
  Mux : xbsIndex_r4/Mux  inputs=2  en=off  latency=0  precision=Full  arith_type=Unsigned  n_bits=16  bin_pt=14  quantization=Truncate  overflow=Wrap  dbl_ovrd=off  block_type=mux
  tag scope: RFA_IQ_RX_ADDR=global, RFA_IQ_RX_DIN=global, RFA_IQ_RX_WE=global
  wires:
  WE/1 -> [RFA_IQ_RX_WE]
  I/Q_32b/1 -> Mux/2, 8LSB+0/1, 8LSB+8/1, 8LSB+16/1, 8LSB+24/1
  Addr/1 -> [RFA_IQ_RX_ADDR]
  Mux/1 -> [RFA_IQ_RX_DIN]
  [RX_BYTE_ORDER] -> Mux/1
  8LSB+0/1 -> Concat/1
  8LSB+8/1 -> Concat/2
  8LSB+16/1 -> Concat/3
  8LSB+24/1 -> Concat/4
  Concat/1 -> Mux/3

== system w3_warplab_buffers/RFA Rx Buffers/RSSI Buffer ==
  Addr : Inport
  RSSI : Inport  Port=2
  WE : Inport  Port=3
  8LSB+0 : xbsIndex_r4/Slice  nbits=8  boolean_output=off  mode=Lower Bit Location + Width  bit1=0  base1=MSB of Input  bit0=0  base0=LSB of Input  dbl_ovrd=off  block_type=slice
  8LSB+16 : xbsIndex_r4/Slice  nbits=8  boolean_output=off  mode=Lower Bit Location + Width  bit1=0  base1=MSB of Input  bit0=16  base0=LSB of Input  dbl_ovrd=off  block_type=slice
  8LSB+24 : xbsIndex_r4/Slice  nbits=8  boolean_output=off  mode=Lower Bit Location + Width  bit1=0  base1=MSB of Input  bit0=24  base0=LSB of Input  dbl_ovrd=off  block_type=slice
  8LSB+8 : xbsIndex_r4/Slice  nbits=8  boolean_output=off  mode=Lower Bit Location + Width  bit1=0  base1=MSB of Input  bit0=8  base0=LSB of Input  dbl_ovrd=off  block_type=slice
  BIT[2] : xbsIndex_r4/Slice  nbits=1  boolean_output=on  mode=Lower Bit Location + Width  bit1=0  base1=MSB of Input  bit0=2  base0=LSB of Input  dbl_ovrd=off  block_type=slice
      settings: infoedit="Extracts a given range of bits from each input sample and presents it at the output.  The output type is ordinarily unsigned with binary point at zero, but can be Boolean when the slice is one bit wide.<P><P>Hardware notes: In hardware this block costs nothing."  block_version=8.2
  Concat : xbsIndex_r4/Concat  num_inputs=2  dbl_ovrd=off  block_type=concat
      settings: block_version=10.1.2
  Concat1 : xbsIndex_r4/Concat  num_inputs=4  dbl_ovrd=off  block_type=concat
  Convert : xbsIndex_r4/Convert  gui_display_data_type=Fixed-point  arith_type=Unsigned  n_bits=16  bin_pt=0  float_type=Single  exp_bits=8  fraction_bits=24  quantization=Truncate  overflow=Wrap  en=off  latency=0  dbl_ovrd=off  pipeline=off  block_type=convert
      settings: block_version=8.2
  Inverter : xbsIndex_r4/Inverter  en=off  latency=0  dbl_ovrd=off  block_type=inv
      settings: block_version=10.1.2
  LSB + 3 : xbsIndex_r4/Slice  nbits=ceil(log2(NumSamps_Rx_RSSI))-1  boolean_output=off  mode=Lower Bit Location + Width  bit1=0  base1=LSB of Input  bit0=3  base0=LSB of Input  dbl_ovrd=off  block_type=slice
      settings: block_version=8.2
  Mux : xbsIndex_r4/Mux  inputs=2  en=off  latency=0  precision=Full  arith_type=Unsigned  n_bits=16  bin_pt=14  quantization=Truncate  overflow=Wrap  dbl_ovrd=off  block_type=mux
  Register : xbsIndex_r4/Register  init=0  rst=off  en=on  dbl_ovrd=off  block_type=register
      settings: block_version=10.1.2
  Reinterpret1 : xbsIndex_r4/Reinterpret  force_arith_type=on  arith_type=Unsigned  force_bin_pt=on  bin_pt=0  block_type=reinterpret
      settings: infoedit="Changes signal type without altering the binary representation.   You can changed the signal between signed and unsigned, and relocate the binary point.<P><P>Hardware notes: In hardware this block costs nothing.<P><P>Example:  Suppose the input is 6 bits wide, signed, with 2 fractional bits, and the output is forced to unsigned with 0 fractional bits.  Then an input of -2.0 (1110.00 in binary 2's complement) becomes an output of 56 (111000 in binary)."  block_version=9.1.01
  tag scope: RFA_RSSI=global, RFA_RSSI_ADDR=global, RFA_RSSI_DIN=global, RFA_RSSI_WE=global
  wires:
  RSSI/1 -> [RFA_RSSI], Reinterpret1/1
  Convert/1 -> Register/1, Concat/2
  Addr/1 -> BIT[2]/1, LSB + 3/1
  Reinterpret1/1 -> Convert/1
  Concat/1 -> 8LSB+0/1, 8LSB+8/1, 8LSB+16/1, 8LSB+24/1, Mux/2
  BIT[2]/1 -> Inverter/1
  LSB + 3/1 -> [RFA_RSSI_ADDR]
  Register/1 -> Concat/1
  Inverter/1 -> Register/2
  [RX_BYTE_ORDER] -> Mux/1
  8LSB+0/1 -> Concat1/1
  8LSB+8/1 -> Concat1/2
  8LSB+16/1 -> Concat1/3
  8LSB+24/1 -> Concat1/4
  Concat1/1 -> Mux/3
  Mux/1 -> [RFA_RSSI_DIN]
  WE/1 -> [RFA_RSSI_WE]
